simulink model "windEmulatorStep4_WECSim"  (R2025b)
settings: Solver=ode14x  StartTime=0  StopTime=400  FixedStep=Ts  MaxStep=0.01  RelTol=1e-3
values from neighbouring files (symbols this model uses):
  A = 1.0    (= 1)    [initStep4.m]
  absEncoderCountsToRad = 1/2^20*2*pi    (= 5.99211245268e-06)    [initStep4.m]
  acs800CtrlStruct =     [windEmulatorBusDefs.mat]
  acs800DcBusVoltsScaling = 1    [initStep4.m]
  acs800FreqScaling = 1/100    (= 0.01)    [initStep4.m]
  acs800PowerScaling = Gen_PowerScaling    (= 14.9109)    [initStep4.m]
  acs800SignalStruct =     [windEmulatorBusDefs.mat]
  acs800SpeedNomEng = 1500    [initStep4.m]
  acs800SpeedNomFb = 20000    [initStep4.m]
  acs800SpeedScaling = 1500/20000    (= 0.075)    [initStep4.m]
  acs800TempScaling = 1/10    (= 0.1)    [initStep4.m]
  acs800TorqueNomEng = 100    [initStep4.m]
  acs800TorqueNomFb = 10000    [initStep4.m]
  acs800TorqueScaling = acs800TorqueRating/10000    (= 0.008035933)    [initStep4.m]
  acs880CtrlStruct =     [windEmulatorBusDefs.mat]
  acs880FreqScaling = 60/20000    (= 0.003)    [initStep4.m]
  acs880MotorCurrentScaling = 100/10000    (= 0.01)    [initStep4.m]
  acs880MotorVoltsScaling = 1    [initStep4.m]
  acs880PowerScaling = 100*hp2W/10000    (= 7.457)    [initStep4.m]
  acs880RatedTorque = 80.494    [initStep4.m]
  acs880RateLimFalling = -10000    [initStep4.m]
  acs880RateLimRising = 10000    [initStep4.m]
  acs880SetpointLimLower = -0.975*acs880RatedTorque    (= -78.48165)    [initStep4.m]
  acs880SetpointLimUpper = 0.975*acs880RatedTorque    (= 78.48165)    [initStep4.m]
  acs880SignalStruct =     [windEmulatorBusDefs.mat]
  acs880SpeedPILimLo = -0.975*acs880RatedTorque    (= -78.48165)    [initStep4.m]
  acs880SpeedPILimUp = 0.975*acs880RatedTorque    (= 78.48165)    [initStep4.m]
  acs880SpeedScaling = 2000/20000    (= 0.1)    [initStep4.m]
  acs880TorqueFieldbusScale = 10000    [initStep4.m]
  acs880TorqueScaling = acs880RatedTorque/acs880TorqueFieldbusScale    (= 0.0080494)    [initStep4.m]
  acs880TorqueSetpointScaling = 100    [initStep4.m]
  bar2pa = 1e5    (= 100000)    [initStep4.m]
  belowMinPGain = 1/200    (= 0.005)    [initStep4.m]
  ctrlModeTorque = logical(true)    [init.m]    (also in initStep1.m; initStep2.m; initStep3.m; initStep4.m)
  ctrlSignal1 = squeeze(hptoSignalsData.Values.ctrlSignal1.Data)    [postProcessingStep2.m]
  ctrlSignal2 = squeeze(hptoSignalsData.Values.ctrlSignal2.Data)    [postProcessingStep2.m]
  deadBandController = boolean(false)    [initStep4.m]
  deadbandTorqueSlewRate = 300    [initStep4.m]
  Dm_max = 40    [initStep4.m]
  EffMechMax = 0.93    [initStep4.m]
  EffMechMin = 0.79    [initStep4.m]
  excForce_N = squeeze(hptoCtrlData.Values.excForce_N.Data)    [postProcessingStep2.m]
  expCtrlStruct =     [windEmulatorBusDefs.mat]
  FactorEff = psi2pa*cc2m3*(1/rev2rad)    (= 0.00109733470463)    [initStep4.m]
  fromFileSpeedSlewRate = 250    [initStep4.m]
  fromFileTorqueSlewRate = 25    [initStep4.m]
  futekTorqueScale = -1/(2^31)*10/5*100    (= -9.31322574615e-08)    [initStep4.m]
  genMaxTorque = 0.8*ratedTorque    (= 64.3952)    [initStep3.m]    (also in initStep4.m = 78.48165)
  genTorqueCmd_Nm = squeeze(hptoSignalsData.Values.genTorqueCmd_Nm.Data)    [postProcessingStep2.m]
  hbmCtScale = 1/1.5    (= 0.666666666667)    [initStep4.m]
  hbmPowerStruct =     [windEmulatorBusDefs.mat]
  hptoCtrlStruct =     [windEmulatorBusDefs.mat]
  hptoSignalStruct =     [windEmulatorBusDefs.mat]
  invPowerStruct =     [windEmulatorBusDefs.mat]
  lpm2m3ps = 1/m3ps2lpm    (= 1.66666666667e-05)    [initStep4.m]
  minPressureRef_psi = 1000    [initStep4.m]
  minTorqueRef_Nm = (minPressureRef_psi*psi2pa)*(Dm_max*cc2m3*(1/rev2rad))    (= 43.8933881851)    [initStep4.m]
  motorSpeed_rpm = squeeze(acs880SignalsData.Values.motorSpeed_rpm.Data)    [postProcessingStep2.m]
  nPreDrop = 2900    [initStep4.m]
  nPreDropMin = 725    [initStep4.m]
  psi2bar = 1/bar2psi    (= 0.0689475729318)    [initStep4.m]
  radps2rpm = 60/(2*pi)    (= 9.54929658551)    [initStep2.m]    (also in initStep4.m)
  rpm2radps = 2*pi/60    (= 0.10471975512)    [initStep4.m]
  runCounter = squeeze(hptoCtrlData.Values.runCounter.Data)    [postProcessingStep2.m]
  shaftSignalStruct =     [windEmulatorBusDefs.mat]
  sidCtrlStruct =     [windEmulatorBusDefs.mat]
  sidDataCaseCounter = sidData.experimentData.count    [initStep4.m]
  sidDataSpeed_rpm = sidData.experimentData.wShaft_rpm    [initStep4.m]
  sidDataTorque_Nm = sidData.experimentData.torqueShaft_Nm    [initStep4.m]
  sidInfoStruct =     [windEmulatorBusDefs.mat]
  T = 4    [initStep4.m]
  targetOmega = 2000/60*2*pi    (= 209.439510239)    [initStep2.m]    (also in initStep3.m; initStep4.m)
  time = hptoCtrlData.Values.runCounter.Time    [postProcessingStep2.m]
  TorqueLoadMax = 75    [initStep4.m]
  Ts = 1/250    (= 0.004)    [initStep4.m]
undefined symbols (not defined in the file or in its folder): absEncoderCounts, absEncoderPosition_rad, absEncoderSpeed_rpm, absEncoderStatus1, absEncoderStatus2, absEncoderTurns, accVolHP, acs800Torque_Nm, acs800TorqueSetpoint_Nm, acs880SpeedSetpoint_rpm, acs880Torque_Nm, body, constraint, crankLength, ctrlWord, dcBusVoltage_V, DiscIntNeverNeededParam, Dmax, excShaftSpeed_rpm, excShaftTorque_Nm, expType, expTypeEnum, frequency_Hz, fromFileCaseCounter, genPumpFlow_lpm, genShaftSpeed_rpm, genShaftSpeedRef, genSpeedActual, hmOutputShafTorque_Nm, iGainGen, m3persecond2lpm, motorCurrent_A, motorTorque_Nm, motorVoltage_V, offsetLength, pa2psi, pGainGen, pressure_bar, PressureControl, pto, radsec2rpm, ramp, resetHilIntegrator, resetSidIntegrator, rodLength, runHil, runSid, shaftPower_W, sidType, sidTypeEnum, SpeedControl, speedCtrlReset, speedRef_rpm, state, statusWord, stepCounter, temperature, torqueActual_Nm, TorqueInputControl, torqueSetpoint_Nm ... (+1)
libraries: slrealtimeethercatlib x118, fl_lib x81, nesl_utility x45, sh_lib x18, slrealtimeloglib x13, dspstat3 x5, slpidlib x4, simulink_extras x4, cstblocks x3, dspindex x3, WECSim_Lib_Body_Elements x2, simulink x2
(part 5 of 6)

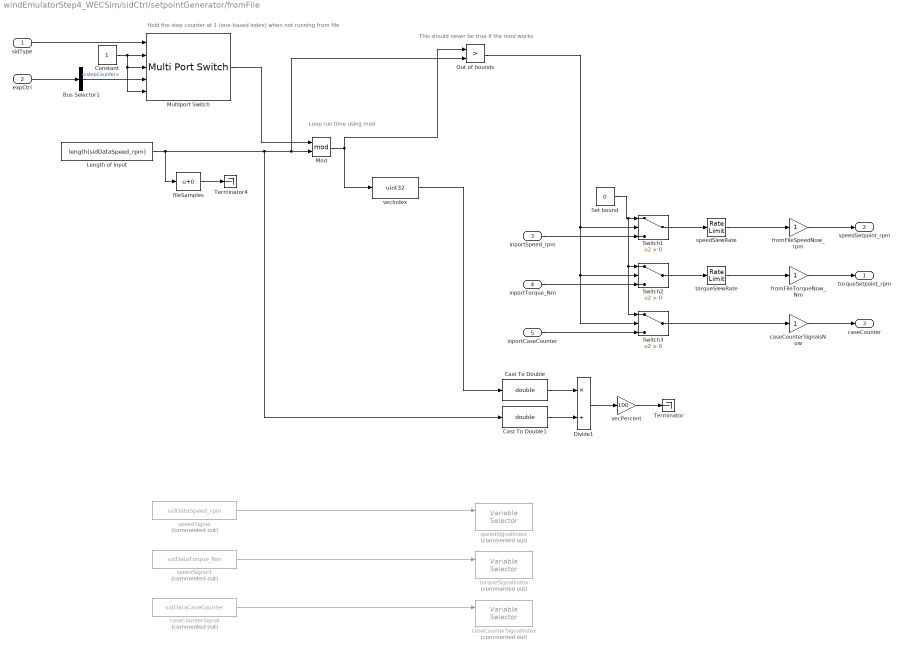
== system windEmulatorStep4_WECSim/sidCtrl/setpointGenerator/fromFile ==
  note: Hold the step counter at 1 (one-based index) when not running from file
  note: This should never be true if the mod works
  note: Loop run time using mod
  sidType : Inport  OutDataTypeStr=Enum: sidTypeEnum
  expCtrl : Inport  Port=2  OutDataTypeStr=Bus: expCtrlBus
  inportSpeed_rpm : Inport  Port=3
  inportTorque_Nm : Inport  Port=4
  inportCaseCounter : Inport  Port=5
  Bus Selector1 : BusSelector  OutputSignals=stepCounter
  Cast To Double : DataTypeConversion  OutDataTypeStr=double  SaturateOnIntegerOverflow=off  RndMeth=Floor
  Cast To Double1 : DataTypeConversion  OutDataTypeStr=double  SaturateOnIntegerOverflow=off  RndMeth=Floor
  Constant : Constant  OutDataTypeStr=uint32
  Divide1 : Product  Inputs=*/
  Length of input : Constant  Value=length(sidDataSpeed_rpm)  OutDataTypeStr=uint32
  Mod : Math  Operator=mod
  Multiport Switch : MultiPortSwitch  DataPortOrder=Specify indices  DataPortIndices={sidTypeEnum.off,sidTypeEnum.manual,sidTypeEnum.fromFile}  DataPortForDefault=Additional data port  SaturateOnIntegerOverflow=off  InputSameDT=off
  Out of bounds : RelationalOperator  Operator=>  OutDataTypeStr=boolean  RndMeth=Simplest  InputSameDT=off
  Set bound : Constant  Value=0
  Switch1 : Switch  Criteria=u2 > Threshold  SaturateOnIntegerOverflow=off  InputSameDT=off
  Switch2 : Switch  Criteria=u2 > Threshold  SaturateOnIntegerOverflow=off  InputSameDT=off
  Switch3 : Switch  Criteria=u2 > Threshold  SaturateOnIntegerOverflow=off  InputSameDT=off
  Terminator : Terminator
  Terminator4 : Terminator
  caseCounterSignal : Constant  Commented=on  Value=sidDataCaseCounter
  caseCounterSignalIndex : dspindex/Variable Selector  Commented=on  NumInputs=1  rowsOrCols=Columns  IdxMode=Variable  Elements=[1 3]  ZerOneIdxMode=One-based  errmode=Clip and Warn  FillMode=on  FillValues=0
  caseCounterSignalsNow : Gain
  fileSamples : Bias  SaturateOnIntegerOverflow=off
  fromFileSpeedNow_rpm : Gain
  fromFileTorqueNow_Nm : Gain
  speedSignal : Constant  Commented=on  Value=sidDataSpeed_rpm
  speedSignal1 : Constant  Commented=on  Value=sidDataTorque_Nm
  speedSignalIndex : dspindex/Variable Selector  Commented=on  NumInputs=1  rowsOrCols=Columns  IdxMode=Variable  Elements=[1 3]  ZerOneIdxMode=One-based  errmode=Clip and Warn  FillMode=on  FillValues=0
  speedSlewRate : RateLimiter  RisingSlewLimit=fromFileSpeedSlewRate  FallingSlewLimit=-fromFileSpeedSlewRate  SampleTimeMode=inherited
  torqueSignalIndex : dspindex/Variable Selector  Commented=on  NumInputs=1  rowsOrCols=Columns  IdxMode=Variable  Elements=[1 3]  ZerOneIdxMode=One-based  errmode=Clip and Warn  FillMode=on  FillValues=0
  torqueSlewRate : RateLimiter  RisingSlewLimit=fromFileTorqueSlewRate  FallingSlewLimit=-fromFileTorqueSlewRate  SampleTimeMode=inherited
  vecIndex : DataTypeConversion  OutDataTypeStr=uint32  SaturateOnIntegerOverflow=off  RndMeth=Floor
  vecPercent : Gain  Gain=100
  torqueSetpoint_rpm : Outport
  speedSetpoint_rpm : Outport  Port=2
  caseCounter : Outport  Port=3
  wires:
  vecPercent/1 -> Terminator/1
  Cast To Double/1 -> Divide1/1
  Length of input/1 -> Cast To Double1/1, Out of bounds/2, Mod/2, fileSamples/1
  fromFileTorqueNow_Nm/1 -> torqueSetpoint_rpm/1
  speedSignal/1 -> speedSignalIndex/1
  Out of bounds/1 -> Switch3/2, Switch2/2, Switch1/2
  torqueSlewRate/1 -> fromFileTorqueNow_Nm/1
  caseCounterSignal/1 -> caseCounterSignalIndex/1
  Switch2/1 -> torqueSlewRate/1
  speedSlewRate/1 -> fromFileSpeedNow_rpm/1
  vecIndex/1 -> Cast To Double/1
  Set bound/1 -> Switch2/1, Switch3/1, Switch1/1
  Switch1/1 -> speedSlewRate/1
  Mod/1 -> vecIndex/1, Out of bounds/1
  fileSamples/1 -> Terminator4/1
  Divide1/1 -> vecPercent/1
  caseCounterSignalsNow/1 -> caseCounter/1
  Switch3/1 -> caseCounterSignalsNow/1
  fromFileSpeedNow_rpm/1 -> speedSetpoint_rpm/1
  Cast To Double1/1 -> Divide1/2
  expCtrl/1 -> Bus Selector1/1
  speedSignal1/1 -> torqueSignalIndex/1
  sidType/1 -> Multiport Switch/1
  Bus Selector1/1 -> Multiport Switch/4  "<stepCounter>"
  Multiport Switch/1 -> Mod/1
  Constant/1 -> Multiport Switch/5, Multiport Switch/3, Multiport Switch/2
  inportSpeed_rpm/1 -> Switch1/3
  inportTorque_Nm/1 -> Switch2/3
  inportCaseCounter/1 -> Switch3/3

== system windEmulatorStep4_WECSim/hptoSim/WECSimModel/Subsystem/Angular to Linear Velocity ==
  angPos : Inport
  angVel : Inport  Port=2
  Add1 : Sum  Inputs=+-
  Add2 : Sum  Inputs=+-
  Add5 : Sum  Inputs=+-
  Add7 : Sum
  Constant1 : Constant  Value=rodLength
  Constant{2,5,8..9} (4 alike) : Constant  Value=crankLength
  Constant3 : Constant  Value=offsetLength
  Constant6 : Constant  Value=offsetLength
  Divide1 : Product  Inputs=*/
  Math Function1 : Math  Operator=square  SignedPower=on
  Math Function2 : Math  Operator=square  SignedPower=on
  Product1 : Product  Inputs=**
  Product5 : Product  Inputs=**
  Product6 : Product  Inputs=***
  Product8 : Product  Inputs=***
  Product9 : Product  Inputs=**
  Sqrt2 : Sqrt
  Trigonometric Function1 : Trigonometry  Operator=cos
  Trigonometric Function3 : Trigonometry  Operator=cos
  Trigonometric Function4 : Trigonometry  Operator=cos
  Trigonometric Function6 : Trigonometry
  linearVel : Outport
  wires:
  Math Function2/1 -> Add1/1
  Divide1/1 -> Add7/2
  Product8/1 -> Divide1/1
  Sqrt2/1 -> Divide1/2
  Math Function1/1 -> Add1/2
  Constant1/1 -> Math Function2/1
  Constant3/1 -> Add2/2
  Product1/1 -> Add2/1
  Trigonometric Function1/1 -> Product1/2
  Constant2/1 -> Product1/1
  Add1/1 -> Sqrt2/1
  Add2/1 -> Math Function1/1
  angPos/1 -> Trigonometric Function4/1, Trigonometric Function3/1, Trigonometric Function6/1, Trigonometric Function1/1
  Product9/1 -> Product8/3
  Add5/1 -> Product8/2
  angVel/1 -> Product6/3, Product8/1
  Trigonometric Function6/1 -> Product9/2
  Constant9/1 -> Product9/1
  Constant6/1 -> Add5/2
  Product5/1 -> Add5/1
  Trigonometric Function3/1 -> Product5/2
  Constant5/1 -> Product5/1
  Product6/1 -> Add7/1
  Constant8/1 -> Product6/1
  Trigonometric Function4/1 -> Product6/2
  Add7/1 -> linearVel/1

== system windEmulatorStep4_WECSim/hptoSim/WECSimModel/Subsystem/FlowSensor1 ==
  Gain : Gain  Gain=m3persecond2lpm
  Hydraulic Flow Rate Sensor : fl_lib/Hydraulic/Hydraulic Sensors/Hydraulic Flow Rate Sensor
  PS Terminator : fl_lib/Physical Signals/Sinks/PS Terminator
  PS-Simulink Converter2 : nesl_utility/PS-Simulink Converter  PhysicalDomain=network_engine_domain  SubClassName=ps_output  LeftPortType=input  RightPortType=output  PseudoPeriodic=off  Frequencies=[]  VectorFormat=inherit  Unit=inherit  AffineConversion=off
  Terminator : Terminator
  B : PMIOPort  Side=Right
  A : PMIOPort  Port=2  Side=Left
  wires:
  PS-Simulink Converter2/1 -> Gain/1
  Gain/1 -> Terminator/1  "flowRateHCB"
  connections:
  Hydraulic Flow Rate Sensor/LConn1 -- A/RConn1
  PS Terminator/LConn1 -- Hydraulic Flow Rate Sensor/RConn3
  PS-Simulink Converter2/LConn1 -- Hydraulic Flow Rate Sensor/RConn1
  Hydraulic Flow Rate Sensor/RConn2 -- B/RConn1

== system windEmulatorStep4_WECSim/hptoSim/WECSimModel/Subsystem/FlowSensor10 ==
  Gain : Gain  Gain=m3persecond2lpm
  Hydraulic Flow Rate Sensor : fl_lib/Hydraulic/Hydraulic Sensors/Hydraulic Flow Rate Sensor
  PS Terminator : fl_lib/Physical Signals/Sinks/PS Terminator
  PS-Simulink Converter2 : nesl_utility/PS-Simulink Converter  PhysicalDomain=network_engine_domain  SubClassName=ps_output  LeftPortType=input  RightPortType=output  PseudoPeriodic=off  Frequencies=[]  VectorFormat=inherit  Unit=inherit  AffineConversion=off
  Terminator : Terminator
  B : PMIOPort  Side=Right
  A : PMIOPort  Port=2  Side=Left
  wires:
  PS-Simulink Converter2/1 -> Gain/1
  Gain/1 -> Terminator/1  "flowRateCV4"
  connections:
  Hydraulic Flow Rate Sensor/LConn1 -- A/RConn1
  PS Terminator/LConn1 -- Hydraulic Flow Rate Sensor/RConn3
  PS-Simulink Converter2/LConn1 -- Hydraulic Flow Rate Sensor/RConn1
  Hydraulic Flow Rate Sensor/RConn2 -- B/RConn1

== system windEmulatorStep4_WECSim/hptoSim/WECSimModel/Subsystem/FlowSensor13 ==
  Gain : Gain  Gain=m3persecond2lpm
  Hydraulic Flow Rate Sensor : fl_lib/Hydraulic/Hydraulic Sensors/Hydraulic Flow Rate Sensor
  PS Terminator : fl_lib/Physical Signals/Sinks/PS Terminator
  PS-Simulink Converter2 : nesl_utility/PS-Simulink Converter  PhysicalDomain=network_engine_domain  SubClassName=ps_output  LeftPortType=input  RightPortType=output  PseudoPeriodic=off  Frequencies=[]  VectorFormat=inherit  Unit=inherit  AffineConversion=off
  Terminator : Terminator
  B : PMIOPort  Side=Right
  A : PMIOPort  Port=2  Side=Left
  wires:
  PS-Simulink Converter2/1 -> Gain/1
  Gain/1 -> Terminator/1  "flowRateCV1"
  connections:
  Hydraulic Flow Rate Sensor/LConn1 -- A/RConn1
  PS Terminator/LConn1 -- Hydraulic Flow Rate Sensor/RConn3
  PS-Simulink Converter2/LConn1 -- Hydraulic Flow Rate Sensor/RConn1
  Hydraulic Flow Rate Sensor/RConn2 -- B/RConn1

== system windEmulatorStep4_WECSim/hptoSim/WECSimModel/Subsystem/FlowSensor16 ==
  Gain : Gain  Gain=m3persecond2lpm
  Hydraulic Flow Rate Sensor : fl_lib/Hydraulic/Hydraulic Sensors/Hydraulic Flow Rate Sensor
  PS Terminator : fl_lib/Physical Signals/Sinks/PS Terminator
  PS-Simulink Converter2 : nesl_utility/PS-Simulink Converter  PhysicalDomain=network_engine_domain  SubClassName=ps_output  LeftPortType=input  RightPortType=output  PseudoPeriodic=off  Frequencies=[]  VectorFormat=inherit  Unit=inherit  AffineConversion=off
  Terminator : Terminator
  B : PMIOPort  Side=Right
  A : PMIOPort  Port=2  Side=Left
  wires:
  PS-Simulink Converter2/1 -> Gain/1
  Gain/1 -> Terminator/1  "flowRateCV3"
  connections:
  Hydraulic Flow Rate Sensor/LConn1 -- A/RConn1
  PS Terminator/LConn1 -- Hydraulic Flow Rate Sensor/RConn3
  PS-Simulink Converter2/LConn1 -- Hydraulic Flow Rate Sensor/RConn1
  Hydraulic Flow Rate Sensor/RConn2 -- B/RConn1

== system windEmulatorStep4_WECSim/hptoSim/WECSimModel/Subsystem/FlowSensor2 ==
  Gain : Gain  Gain=m3persecond2lpm
  Hydraulic Flow Rate Sensor : fl_lib/Hydraulic/Hydraulic Sensors/Hydraulic Flow Rate Sensor
  PS Terminator : fl_lib/Physical Signals/Sinks/PS Terminator
  PS-Simulink Converter2 : nesl_utility/PS-Simulink Converter  PhysicalDomain=network_engine_domain  SubClassName=ps_output  LeftPortType=input  RightPortType=output  PseudoPeriodic=off  Frequencies=[]  VectorFormat=inherit  Unit=inherit  AffineConversion=off
  Terminator : Terminator
  B : PMIOPort  Side=Right
  A : PMIOPort  Port=2  Side=Left
  wires:
  PS-Simulink Converter2/1 -> Gain/1
  Gain/1 -> Terminator/1  "flowRateHCA"
  connections:
  Hydraulic Flow Rate Sensor/LConn1 -- A/RConn1
  PS Terminator/LConn1 -- Hydraulic Flow Rate Sensor/RConn3
  PS-Simulink Converter2/LConn1 -- Hydraulic Flow Rate Sensor/RConn1
  Hydraulic Flow Rate Sensor/RConn2 -- B/RConn1

== system windEmulatorStep4_WECSim/hptoSim/WECSimModel/Subsystem/FlowSensor3 ==
  Gain : Gain  Gain=m3persecond2lpm
  Hydraulic Flow Rate Sensor : fl_lib/Hydraulic/Hydraulic Sensors/Hydraulic Flow Rate Sensor
  PS Terminator : fl_lib/Physical Signals/Sinks/PS Terminator
  PS-Simulink Converter2 : nesl_utility/PS-Simulink Converter  PhysicalDomain=network_engine_domain  SubClassName=ps_output  LeftPortType=input  RightPortType=output  PseudoPeriodic=off  Frequencies=[]  VectorFormat=inherit  Unit=inherit  AffineConversion=off
  Terminator : Terminator
  B : PMIOPort  Side=Right
  A : PMIOPort  Port=2  Side=Left
  wires:
  PS-Simulink Converter2/1 -> Gain/1
  Gain/1 -> Terminator/1  "flowRateC"
  connections:
  Hydraulic Flow Rate Sensor/LConn1 -- A/RConn1
  PS Terminator/LConn1 -- Hydraulic Flow Rate Sensor/RConn3
  PS-Simulink Converter2/LConn1 -- Hydraulic Flow Rate Sensor/RConn1
  Hydraulic Flow Rate Sensor/RConn2 -- B/RConn1

== system windEmulatorStep4_WECSim/hptoSim/WECSimModel/Subsystem/FlowSensor4 ==
  Gain : Gain  Gain=m3persecond2lpm
  Hydraulic Flow Rate Sensor : fl_lib/Hydraulic/Hydraulic Sensors/Hydraulic Flow Rate Sensor
  PS Terminator : fl_lib/Physical Signals/Sinks/PS Terminator
  PS-Simulink Converter2 : nesl_utility/PS-Simulink Converter  PhysicalDomain=network_engine_domain  SubClassName=ps_output  LeftPortType=input  RightPortType=output  PseudoPeriodic=off  Frequencies=[]  VectorFormat=inherit  Unit=inherit  AffineConversion=off
  Terminator : Terminator
  B : PMIOPort  Side=Right
  A : PMIOPort  Port=2  Side=Left
  wires:
  PS-Simulink Converter2/1 -> Gain/1
  Gain/1 -> Terminator/1  "flowRateAccHP"
  connections:
  Hydraulic Flow Rate Sensor/LConn1 -- A/RConn1
  PS Terminator/LConn1 -- Hydraulic Flow Rate Sensor/RConn3
  PS-Simulink Converter2/LConn1 -- Hydraulic Flow Rate Sensor/RConn1
  Hydraulic Flow Rate Sensor/RConn2 -- B/RConn1

== system windEmulatorStep4_WECSim/hptoSim/WECSimModel/Subsystem/FlowSensor5 ==
  Gain : Gain  Gain=m3persecond2lpm
  Hydraulic Flow Rate Sensor : fl_lib/Hydraulic/Hydraulic Sensors/Hydraulic Flow Rate Sensor
  PS Terminator : fl_lib/Physical Signals/Sinks/PS Terminator
  PS-Simulink Converter2 : nesl_utility/PS-Simulink Converter  PhysicalDomain=network_engine_domain  SubClassName=ps_output  LeftPortType=input  RightPortType=output  PseudoPeriodic=off  Frequencies=[]  VectorFormat=inherit  Unit=inherit  AffineConversion=off
  Terminator : Terminator
  B : PMIOPort  Side=Right
  A : PMIOPort  Port=2  Side=Left
  wires:
  PS-Simulink Converter2/1 -> Gain/1
  Gain/1 -> Terminator/1  "flowRateHMin"
  connections:
  Hydraulic Flow Rate Sensor/LConn1 -- A/RConn1
  PS Terminator/LConn1 -- Hydraulic Flow Rate Sensor/RConn3
  PS-Simulink Converter2/LConn1 -- Hydraulic Flow Rate Sensor/RConn1
  Hydraulic Flow Rate Sensor/RConn2 -- B/RConn1

== system windEmulatorStep4_WECSim/hptoSim/WECSimModel/Subsystem/FlowSensor6 ==
  Gain : Gain  Gain=m3persecond2lpm
  Hydraulic Flow Rate Sensor : fl_lib/Hydraulic/Hydraulic Sensors/Hydraulic Flow Rate Sensor
  PS Terminator : fl_lib/Physical Signals/Sinks/PS Terminator
  PS-Simulink Converter2 : nesl_utility/PS-Simulink Converter  PhysicalDomain=network_engine_domain  SubClassName=ps_output  LeftPortType=input  RightPortType=output  PseudoPeriodic=off  Frequencies=[]  VectorFormat=inherit  Unit=inherit  AffineConversion=off
  Terminator : Terminator
  B : PMIOPort  Side=Right
  A : PMIOPort  Port=2  Side=Left
  wires:
  PS-Simulink Converter2/1 -> Gain/1
  Gain/1 -> Terminator/1  "flowRateHMout"
  connections:
  Hydraulic Flow Rate Sensor/LConn1 -- A/RConn1
  PS Terminator/LConn1 -- Hydraulic Flow Rate Sensor/RConn3
  PS-Simulink Converter2/LConn1 -- Hydraulic Flow Rate Sensor/RConn1
  Hydraulic Flow Rate Sensor/RConn2 -- B/RConn1

== system windEmulatorStep4_WECSim/hptoSim/WECSimModel/Subsystem/FlowSensor7 ==
  Gain : Gain  Gain=m3persecond2lpm
  Hydraulic Flow Rate Sensor : fl_lib/Hydraulic/Hydraulic Sensors/Hydraulic Flow Rate Sensor
  PS Terminator : fl_lib/Physical Signals/Sinks/PS Terminator
  PS-Simulink Converter2 : nesl_utility/PS-Simulink Converter  PhysicalDomain=network_engine_domain  SubClassName=ps_output  LeftPortType=input  RightPortType=output  PseudoPeriodic=off  Frequencies=[]  VectorFormat=inherit  Unit=inherit  AffineConversion=off
  Terminator : Terminator
  B : PMIOPort  Side=Right
  A : PMIOPort  Port=2  Side=Left
  wires:
  PS-Simulink Converter2/1 -> Gain/1
  Gain/1 -> Terminator/1  "flowRateAccLP"
  connections:
  Hydraulic Flow Rate Sensor/LConn1 -- A/RConn1
  PS Terminator/LConn1 -- Hydraulic Flow Rate Sensor/RConn3
  PS-Simulink Converter2/LConn1 -- Hydraulic Flow Rate Sensor/RConn1
  Hydraulic Flow Rate Sensor/RConn2 -- B/RConn1

== system windEmulatorStep4_WECSim/hptoSim/WECSimModel/Subsystem/FlowSensor8 ==
  Gain : Gain  Gain=m3persecond2lpm
  Hydraulic Flow Rate Sensor : fl_lib/Hydraulic/Hydraulic Sensors/Hydraulic Flow Rate Sensor
  PS Terminator : fl_lib/Physical Signals/Sinks/PS Terminator
  PS-Simulink Converter2 : nesl_utility/PS-Simulink Converter  PhysicalDomain=network_engine_domain  SubClassName=ps_output  LeftPortType=input  RightPortType=output  PseudoPeriodic=off  Frequencies=[]  VectorFormat=inherit  Unit=inherit  AffineConversion=off
  Terminator : Terminator
  B : PMIOPort  Side=Right
  A : PMIOPort  Port=2  Side=Left
  wires:
  PS-Simulink Converter2/1 -> Gain/1
  Gain/1 -> Terminator/1  "flowRateD"
  connections:
  Hydraulic Flow Rate Sensor/LConn1 -- A/RConn1
  PS Terminator/LConn1 -- Hydraulic Flow Rate Sensor/RConn3
  PS-Simulink Converter2/LConn1 -- Hydraulic Flow Rate Sensor/RConn1
  Hydraulic Flow Rate Sensor/RConn2 -- B/RConn1

== system windEmulatorStep4_WECSim/hptoSim/WECSimModel/Subsystem/FlowSensor9 ==
  Gain : Gain  Gain=m3persecond2lpm
  Hydraulic Flow Rate Sensor : fl_lib/Hydraulic/Hydraulic Sensors/Hydraulic Flow Rate Sensor
  PS Terminator : fl_lib/Physical Signals/Sinks/PS Terminator
  PS-Simulink Converter2 : nesl_utility/PS-Simulink Converter  PhysicalDomain=network_engine_domain  SubClassName=ps_output  LeftPortType=input  RightPortType=output  PseudoPeriodic=off  Frequencies=[]  VectorFormat=inherit  Unit=inherit  AffineConversion=off
  Terminator : Terminator
  B : PMIOPort  Side=Right
  A : PMIOPort  Port=2  Side=Left
  wires:
  PS-Simulink Converter2/1 -> Gain/1
  Gain/1 -> Terminator/1  "flowRateCV2"
  connections:
  Hydraulic Flow Rate Sensor/LConn1 -- A/RConn1
  PS Terminator/LConn1 -- Hydraulic Flow Rate Sensor/RConn3
  PS-Simulink Converter2/LConn1 -- Hydraulic Flow Rate Sensor/RConn1
  Hydraulic Flow Rate Sensor/RConn2 -- B/RConn1

== system windEmulatorStep4_WECSim/hptoSim/WECSimModel/Subsystem/pistonPosition ==
  Ideal Translational Motion Sensor : fl_lib/Mechanical/Mechanical Sensors/Ideal Translational Motion Sensor  reference=foundation.enum.MeasurementReference.difference  acceleration_port=false  velocity_port=true  position_port=true  offset=0 m
  Mechanical Translational Reference1 : fl_lib/Mechanical/Translational Elements/Mechanical Translational Reference
  PS Terminator : fl_lib/Physical Signals/Sinks/PS Terminator
  PS-Simulink Converter : nesl_utility/PS-Simulink Converter  PhysicalDomain=network_engine_domain  SubClassName=ps_output  LeftPortType=input  RightPortType=output  PseudoPeriodic=off  Frequencies=[]  VectorFormat=inherit  Unit=inherit  AffineConversion=off
  PS-Simulink Converter2 : nesl_utility/PS-Simulink Converter  PhysicalDomain=network_engine_domain  SubClassName=ps_output  LeftPortType=input  RightPortType=output  PseudoPeriodic=off  Frequencies=[]  VectorFormat=inherit  Unit=inherit  AffineConversion=off
  Scope : Scope
      settings: ActiveDisplayYMinimum=-0.080911717849368445  ActiveDisplayYMaximum=0.6625292550148727  DataLoggingVariableName=ScopeData5
  Terminator : Terminator
  Conn1 : PMIOPort  Side=Left
  Out1 : Outport
  wires:
  PS-Simulink Converter2/1 -> Scope/1, Terminator/1  "pistonPosition"
  PS-Simulink Converter/1 -> Out1/1
  connections:
  Ideal Translational Motion Sensor/LConn1 -- Conn1/RConn1
  PS Terminator/LConn1 -- PS-Simulink Converter/LConn1 -- Ideal Translational Motion Sensor/RConn2
  PS-Simulink Converter2/LConn1 -- Ideal Translational Motion Sensor/RConn3
  Mechanical Translational Reference1/LConn1 -- Ideal Translational Motion Sensor/RConn1

== system windEmulatorStep4_WECSim/hptoSim/WECSimModel/Subsystem/pressureSensorA ==
  Gain : Gain  Gain=pa2psi
  Hydraulic Pressure Sensor : fl_lib/Hydraulic/Hydraulic Sensors/Hydraulic Pressure Sensor
  Hydraulic Reference : fl_lib/Hydraulic/Hydraulic Elements/Hydraulic Reference
  PS-Simulink Converter2 : nesl_utility/PS-Simulink Converter  PhysicalDomain=network_engine_domain  SubClassName=ps_output  LeftPortType=input  RightPortType=output  PseudoPeriodic=off  Frequencies=[]  VectorFormat=inherit  Unit=inherit  AffineConversion=off
  Scope : Scope
      settings: ActiveDisplayYMinimum=-108.18611715828341  ActiveDisplayYMaximum=973.67505442455092  DataLoggingVariableName=ScopeData4
  Terminator : Terminator
  Conn1 : PMIOPort  Side=Left
  wires:
  Gain/1 -> Scope/1, Terminator/1  "pressureA"
  PS-Simulink Converter2/1 -> Gain/1
  connections:
  PS-Simulink Converter2/LConn1 -- Hydraulic Pressure Sensor/RConn2
  Hydraulic Reference/LConn1 -- Hydraulic Pressure Sensor/RConn1
  Hydraulic Pressure Sensor/LConn1 -- Conn1/RConn1

== system windEmulatorStep4_WECSim/hptoSim/WECSimModel/Subsystem/pressureSensorB ==
  Gain : Gain  Gain=pa2psi
  Hydraulic Pressure Sensor : fl_lib/Hydraulic/Hydraulic Sensors/Hydraulic Pressure Sensor
  Hydraulic Reference : fl_lib/Hydraulic/Hydraulic Elements/Hydraulic Reference
  PS-Simulink Converter2 : nesl_utility/PS-Simulink Converter  PhysicalDomain=network_engine_domain  SubClassName=ps_output  LeftPortType=input  RightPortType=output  PseudoPeriodic=off  Frequencies=[]  VectorFormat=inherit  Unit=inherit  AffineConversion=off
  Scope : Scope
      settings: ActiveDisplayYMinimum=-22.167205478263213  ActiveDisplayYMaximum=1755.5061383660914  DataLoggingVariableName=ScopeData3
  Terminator : Terminator
  Conn1 : PMIOPort  Side=Left
  wires:
  Gain/1 -> Scope/1, Terminator/1  "pressureB"
  PS-Simulink Converter2/1 -> Gain/1
  connections:
  PS-Simulink Converter2/LConn1 -- Hydraulic Pressure Sensor/RConn2
  Hydraulic Reference/LConn1 -- Hydraulic Pressure Sensor/RConn1
  Hydraulic Pressure Sensor/LConn1 -- Conn1/RConn1

== system windEmulatorStep4_WECSim/hptoSim/WECSimModel/Subsystem/pressureSensorC ==
  Gain : Gain  Gain=pa2psi
  Hydraulic Pressure Sensor : fl_lib/Hydraulic/Hydraulic Sensors/Hydraulic Pressure Sensor
  Hydraulic Reference : fl_lib/Hydraulic/Hydraulic Elements/Hydraulic Reference
  PS-Simulink Converter2 : nesl_utility/PS-Simulink Converter  PhysicalDomain=network_engine_domain  SubClassName=ps_output  LeftPortType=input  RightPortType=output  PseudoPeriodic=off  Frequencies=[]  VectorFormat=inherit  Unit=inherit  AffineConversion=off
  Terminator : Terminator
  Conn1 : PMIOPort  Side=Left
  wires:
  Gain/1 -> Terminator/1  "pressureC"
  PS-Simulink Converter2/1 -> Gain/1
  connections:
  PS-Simulink Converter2/LConn1 -- Hydraulic Pressure Sensor/RConn2
  Hydraulic Reference/LConn1 -- Hydraulic Pressure Sensor/RConn1
  Hydraulic Pressure Sensor/LConn1 -- Conn1/RConn1

== system windEmulatorStep4_WECSim/hptoSim/WECSimModel/Subsystem/pressureSensorC1 ==
  Gain : Gain  Gain=pa2psi
  Hydraulic Pressure Sensor : fl_lib/Hydraulic/Hydraulic Sensors/Hydraulic Pressure Sensor
  Hydraulic Reference : fl_lib/Hydraulic/Hydraulic Elements/Hydraulic Reference
  PS-Simulink Converter2 : nesl_utility/PS-Simulink Converter  PhysicalDomain=network_engine_domain  SubClassName=ps_output  LeftPortType=input  RightPortType=output  PseudoPeriodic=off  Frequencies=[]  VectorFormat=inherit  Unit=inherit  AffineConversion=off
  Scope : Scope
      settings: ActiveDisplayYMinimum=129.86941769572641  ActiveDisplayYMaximum=1541.1272657005441  DataLoggingVariableName=ScopeData6
  Terminator : Terminator
  Conn1 : PMIOPort  Side=Left
  wires:
  Gain/1 -> Scope/1, Terminator/1  "pressureHM"
  PS-Simulink Converter2/1 -> Gain/1
  connections:
  PS-Simulink Converter2/LConn1 -- Hydraulic Pressure Sensor/RConn2
  Hydraulic Reference/LConn1 -- Hydraulic Pressure Sensor/RConn1
  Hydraulic Pressure Sensor/LConn1 -- Conn1/RConn1

== system windEmulatorStep4_WECSim/hptoSim/WECSimModel/Subsystem/pressureSensorD ==
  Gain : Gain  Gain=pa2psi
  Hydraulic Pressure Sensor : fl_lib/Hydraulic/Hydraulic Sensors/Hydraulic Pressure Sensor
  Hydraulic Reference : fl_lib/Hydraulic/Hydraulic Elements/Hydraulic Reference
  PS-Simulink Converter2 : nesl_utility/PS-Simulink Converter  PhysicalDomain=network_engine_domain  SubClassName=ps_output  LeftPortType=input  RightPortType=output  PseudoPeriodic=off  Frequencies=[]  VectorFormat=inherit  Unit=inherit  AffineConversion=off
  Scope : Scope
      settings: ActiveDisplayYMinimum=-6.2082719103911472  ActiveDisplayYMaximum=137.72426049135703  DataLoggingVariableName=ScopeData7
  Terminator : Terminator
  Conn1 : PMIOPort  Side=Left
  wires:
  Gain/1 -> Scope/1, Terminator/1  "pressureD"
  PS-Simulink Converter2/1 -> Gain/1
  connections:
  PS-Simulink Converter2/LConn1 -- Hydraulic Pressure Sensor/RConn2
  Hydraulic Reference/LConn1 -- Hydraulic Pressure Sensor/RConn1
  Hydraulic Pressure Sensor/LConn1 -- Conn1/RConn1

== system windEmulatorStep4_WECSim/hptoSim/hptoModel/ControlAlgorithm/ForceToTorque ==
  ActualSignals : Inport
  Bus Selector : BusSelector  OutputSignals=LinearSpeedInput,LinearPositionInput
  Constant2 : Constant  Value=(A*2*pi/T)/targetOmega
  DesiredForce : Subsystem
  Gain : Gain  Gain=-1
  Product2 : Product
  TorqueD : Outport
  wires:
  ActualSignals/1 -> Bus Selector/1
  Product2/1 -> Gain/1
  Constant2/1 -> Product2/2
  Bus Selector/1 -> DesiredForce/1(<LinearSpeedInput>)  "<LinearSpeedInput>"
  Bus Selector/2 -> DesiredForce/2(<LinearPositionInput>)  "<LinearPositionInput>"
  DesiredForce/1(ForceD) -> Product2/1
  Gain/1 -> TorqueD/1

== system windEmulatorStep4_WECSim/hptoSim/hptoModel/ControlAlgorithm/PressureAbovePmin ==
  ActualSignals : Inport
  RefValues : Inport  Port=2
  SpeedControllerReset : Inport  Port=3
  Bus Selector : BusSelector  OutputSignals=TorqueShaftInput,Pressure,wShaft
  Bus Selector1 : BusSelector  OutputSignals=TorqueInputRef,PressureRef,SheftSpeedRef
  PressureControl1 : Subsystem
  SpeedControl1 : Subsystem
  Terminator1 : Terminator
  TorqueControl1 : Subsystem
  ControlSignal1 : Outport
  ControlSignal2 : Outport  Port=2
  ControlTorqueLoad : Outport  Port=3
  wires:
  ActualSignals/1 -> Bus Selector/1
  TorqueControl1/1(ControlSignal1) -> ControlSignal1/1
  Bus Selector/3 -> SpeedControl1/1(ShaftSpeedMotor)  "<wShaft>"
  RefValues/1 -> Bus Selector1/1
  Bus Selector1/1 -> TorqueControl1/1(TorqueRef)  "<TorqueInputRef>"
  Bus Selector1/3 -> SpeedControl1/2(ShaftSpeedRef)  "<SheftSpeedRef>"
  PressureControl1/1(ControlSignal2) -> ControlSignal2/1
  Bus Selector/2 -> PressureControl1/1(ActualPressure)  "<Pressure>"
  Bus Selector/1 -> Terminator1/1  "<TorqueShaftInput>"
  Bus Selector1/2 -> PressureControl1/2(PressureRef)  "<PressureRef>"
  SpeedControl1/1(ContolTorque) -> ControlTorqueLoad/1
  SpeedControllerReset/1 -> SpeedControl1/3(SpeedControllerReset)

== system windEmulatorStep4_WECSim/hptoSim/hptoModel/ControlAlgorithm/PressureBelowPmin ==
  ActualSignals : Inport
  RefValues : Inport  Port=2
  SpeedControllerReset : Inport  Port=3
  Bus Selector : BusSelector  OutputSignals=TorqueShaftInput,Pressure,wShaft
  Bus Selector1 : BusSelector  OutputSignals=TorqueInputRef,PressureRef,SheftSpeedRef
  PressureControl1 : Subsystem
  SpeedControl1 : Subsystem
  TorqueControl1 : Subsystem
  ControlSignal1 : Outport
  ControlSignal2 : Outport  Port=2
  ControlTorqueLoad : Outport  Port=3
  wires:
  ActualSignals/1 -> Bus Selector/1
  Bus Selector/1 -> TorqueControl1/1(ActualTorqueInput)  "<TorqueShaftInput>"
  TorqueControl1/1(ControlSignal1) -> ControlSignal1/1
  PressureControl1/1(ControlSignal2) -> ControlSignal2/1
  Bus Selector/2 -> TorqueControl1/3(Pressure), PressureControl1/1(ActualPressure)  "<Pressure>"
  Bus Selector/3 -> SpeedControl1/1(ShaftSpeedMotor)  "<wShaft>"
  SpeedControl1/1(ContolTorque) -> ControlTorqueLoad/1
  RefValues/1 -> Bus Selector1/1
  Bus Selector1/1 -> TorqueControl1/2(TorqueRef)  "<TorqueInputRef>"
  Bus Selector1/2 -> PressureControl1/2(PressureRef)  "<PressureRef>"
  Bus Selector1/3 -> SpeedControl1/2(ShaftSpeedRef)  "<SheftSpeedRef>"
  SpeedControllerReset/1 -> SpeedControl1/3(SpeedControllerReset)

== system windEmulatorStep4_WECSim/hptoSim/hptoModel/HPTO/ChargeCircuit ==
  note: Pressure compensated charge pump
  Check Valve1 : sh_lib/Valves/Directional Valves/Check Valve  area_max=1e-2 m^2  pres_crack=2 bar  pres_max=4 bar  C_d=0.7  A_leak=1e-12 m^2  lam_spec=1  B_lam=0.999  Re_cr=12  dynamic=0  tau=0.1 s  area_init=1e-12 m^2
      settings: InternalSimscapePortConfiguration="{\"Bottom\":[],\"Left\":[{\"id\":\"A\",\"label\":\"A\",\"type\":\"foundation.hydraulic.hydraulic\"}],\"Right\":[{\"id\":\"B\",\"label\":\"B\",\"type\":\"foundation.hydraulic.hydraulic\"}],\"Top\":[]}"
  Constant1 : Constant  Value=2000*rpm2radps
  Gas-Charged Accumulator2 : sh_lib/Accumulators/Gas-Charged Accumulator  capacity=5e-3 m^3  dead_volume=4e-5 m^3  pr_preload=100 psi  k_sh=1.4  stiff_coeff=1e10 Pa/m^3  penetr_coeff=1e10 Pa*s/m^6  flow_rate_specify=off  flow_rate_priority=None  flow_rate=5e-3 m^3/s  flow_rate_nominal_specify=off  flow_rate_nominal_value=1  flow_rate_nominal_unit=m^3/s  liquid_volume_specify=on  liquid_volume_priority=High  liquid_volume=4.9e-3 m^3  liquid_volume_nominal_specify=off  liquid_volume_nominal_value=1  liquid_volume_nominal_unit=m^3  liquid_pressure_specify=on  liquid_pressure_priority=High  liquid_pressure=400 psi  liquid_pressure_nominal_specify=off  liquid_pressure_nominal_value=1  liquid_pressure_nominal_unit=Pa
      settings: InternalSimscapePortConfiguration="{\"Bottom\":[],\"Left\":[],\"Right\":[{\"id\":\"A\",\"label\":\"A\",\"type\":\"foundation.hydraulic.hydraulic\"}],\"Top\":[]}"
  Ideal Angular Velocity Source : fl_lib/Mechanical/Mechanical Sources/Ideal Angular Velocity Source
  Mechanical Rotational Reference : fl_lib/Mechanical/Rotational Elements/Mechanical Rotational Reference
  Pressure Relief Valve2 : sh_lib/Valves/Pressure Control Valves/Pressure Relief Valve  valve_area_spec=1  p_diff_TLU=[30.15e5 : 15e3 : 31.35e5] Pa  area_TLU=[1 : 1 : 9] .* 1e-5 m^2  area_max=1e-4 m^2  pres_set=30 bar  reg_range=1 bar  C_d=0.7  A_leak=1e-12 m^2  lam_spec=1  B_lam=0.999  Re_cr=12  dynamic=0  tau=0.1 s  area_init=1e-12 m^2
      settings: InternalSimscapePortConfiguration="{\"Bottom\":[],\"Left\":[{\"id\":\"A\",\"label\":\"A\",\"type\":\"foundation.hydraulic.hydraulic\"}],\"Right\":[{\"id\":\"B\",\"label\":\"B\",\"type\":\"foundation.hydraulic.hydraulic\"}],\"Top\":[]}"
  Rate Limiter : RateLimiter  RisingSlewLimit=200  FallingSlewLimit=-200  SampleTimeMode=inherited
  Simulink-PS Converter1 : nesl_utility/Simulink-PS Converter  PhysicalDomain=network_engine_domain  SubClassName=ps_input  LeftPortType=input  RightPortType=output  PseudoPeriodic=off  Frequencies=[]  NoiseDistribution=none  NoiseParameters=[]  Unit=1  AffineConversion=off  FilteringAndDerivatives=provide  SimscapeFilterOrder=1  InputFilterTimeConstant=0.001  UdotUserProvided=0
  Variable-Displacement Pressure-Compensated Pump1 : sh_lib/Pumps and Motors/Variable-Displacement Pressure-Compensated Pump  D_max=0.2 l/rev  pr_set=20 bar  pr_reg=1 bar  efficiency_vol=0.85  efficiency_tot=0.75  pr_nominal=20 bar  w_nominal=1800 rpm  visc_nominal=18 cSt  dens_nominal=950 kg/m^3
      settings: InternalSimscapePortConfiguration="{\"Bottom\":[],\"Left\":[{\"id\":\"S\",\"label\":\"S\",\"type\":\"foundation.mechanical.rotational.rotational\"}],\"Right\":[{\"id\":\"P\",\"label\":\"P\",\"type\":\"foundation.hydraulic.hydraulic\"},{\"id\":\"T\",\"label\":\"T\",\"type\":\"foundation.hydraulic.hydraulic\"}],\"Top\":[]}"
  Conn1 : PMIOPort  Side=Left
  Conn2 : PMIOPort  Port=2  Side=Right
  wires:
  Rate Limiter/1 -> Simulink-PS Converter1/1
  Constant1/1 -> Rate Limiter/1
  connections:
  Variable-Displacement Pressure-Compensated Pump1/RConn2 -- Pressure Relief Valve2/RConn1 -- Conn2/RConn1
  Variable-Displacement Pressure-Compensated Pump1/RConn1 -- Gas-Charged Accumulator2/RConn1 -- Check Valve1/LConn1 -- Pressure Relief Valve2/LConn1
  Simulink-PS Converter1/RConn1 -- Ideal Angular Velocity Source/RConn1
  Ideal Angular Velocity Source/RConn2 -- Mechanical Rotational Reference/LConn1
  Variable-Displacement Pressure-Compensated Pump1/LConn1 -- Ideal Angular Velocity Source/LConn1
  Conn1/RConn1 -- Check Valve1/RConn1

== system windEmulatorStep4_WECSim/hptoSim/hptoModel/HPTO/FlowSensor ==
  Hydraulic Flow Rate Sensor : fl_lib/Hydraulic/Hydraulic Sensors/Hydraulic Flow Rate Sensor
  PS Terminator : fl_lib/Physical Signals/Sinks/PS Terminator
  PS-Simulink Converter : nesl_utility/PS-Simulink Converter  PhysicalDomain=network_engine_domain  SubClassName=ps_output  LeftPortType=input  RightPortType=output  PseudoPeriodic=off  Frequencies=[]  VectorFormat=1-D array  Unit=inherit  AffineConversion=off
  Scope : Scope
  m3toL : Gain  Gain=1000*60
  Qin : PMIOPort  Side=Left
  Qout : PMIOPort  Port=2  Side=Right
  FlowPump1 : Outport
  wires:
  PS-Simulink Converter/1 -> m3toL/1, Scope/1
  m3toL/1 -> FlowPump1/1  "FlowPump1"
  connections:
  PS-Simulink Converter/LConn1 -- Hydraulic Flow Rate Sensor/RConn1
  Hydraulic Flow Rate Sensor/RConn2 -- Qout/RConn1
  PS Terminator/LConn1 -- Hydraulic Flow Rate Sensor/RConn3
  Hydraulic Flow Rate Sensor/LConn1 -- Qin/RConn1

== system windEmulatorStep4_WECSim/hptoSim/hptoModel/HPTO/FlowSensor1 ==
  Gain : Gain  Gain=1000*60
  Hydraulic Flow Rate Sensor : fl_lib/Hydraulic/Hydraulic Sensors/Hydraulic Flow Rate Sensor
  PS Terminator : fl_lib/Physical Signals/Sinks/PS Terminator
  PS-Simulink Converter : nesl_utility/PS-Simulink Converter  PhysicalDomain=network_engine_domain  SubClassName=ps_output  LeftPortType=input  RightPortType=output  PseudoPeriodic=off  Frequencies=[]  VectorFormat=1-D array  Unit=inherit  AffineConversion=off
  Scope : Scope
  Qin : PMIOPort  Side=Left
  Qout : PMIOPort  Port=2  Side=Right
  wires:
  PS-Simulink Converter/1 -> Gain/1
  Gain/1 -> Scope/1  "FlowAccumulator"
  connections:
  PS-Simulink Converter/LConn1 -- Hydraulic Flow Rate Sensor/RConn1
  Hydraulic Flow Rate Sensor/RConn2 -- Qout/RConn1
  PS Terminator/LConn1 -- Hydraulic Flow Rate Sensor/RConn3
  Hydraulic Flow Rate Sensor/LConn1 -- Qin/RConn1

== system windEmulatorStep4_WECSim/hptoSim/hptoModel/HPTO/FlowSensor2 ==
  Gain : Gain  Gain=1000*60
  Hydraulic Flow Rate Sensor : fl_lib/Hydraulic/Hydraulic Sensors/Hydraulic Flow Rate Sensor
  PS Terminator : fl_lib/Physical Signals/Sinks/PS Terminator
  PS-Simulink Converter : nesl_utility/PS-Simulink Converter  PhysicalDomain=network_engine_domain  SubClassName=ps_output  LeftPortType=input  RightPortType=output  PseudoPeriodic=off  Frequencies=[]  VectorFormat=1-D array  Unit=inherit  AffineConversion=off
  Qin : PMIOPort  Side=Left
  Qout : PMIOPort  Port=2  Side=Right
  HMFlow_lpm : Outport
  wires:
  PS-Simulink Converter/1 -> Gain/1
  Gain/1 -> HMFlow_lpm/1  "FlowMotor1"
  connections:
  PS-Simulink Converter/LConn1 -- Hydraulic Flow Rate Sensor/RConn1
  Hydraulic Flow Rate Sensor/RConn2 -- Qout/RConn1
  PS Terminator/LConn1 -- Hydraulic Flow Rate Sensor/RConn3
  Hydraulic Flow Rate Sensor/LConn1 -- Qin/RConn1

== system windEmulatorStep4_WECSim/hptoSim/hptoModel/HPTO/LinearVelInput ==
  Fexc : Inport
  Ideal Force Sensor1 : fl_lib/Mechanical/Mechanical Sensors/Ideal Force Sensor
  PS-Simulink Converter : nesl_utility/PS-Simulink Converter  PhysicalDomain=network_engine_domain  SubClassName=ps_output  LeftPortType=input  RightPortType=output  PseudoPeriodic=off  Frequencies=[]  VectorFormat=1-D array  Unit=inherit  AffineConversion=off
  Subsystem : Subsystem
      settings: PortSchema="{\"entries\":[{\"content\":{\"sides\":[{\"content\":{\"connectorIds\":[\"LConn1\"]},\"type\":\"ConnectorPlacement.EquallySpacedRectSide\",\"uuid\":\"215b7bca-b171-42a0-8110-3ac7d91926b2\"},{\"content\":{\"connectorIds\":[\"RConn1\"],\"side\":\"RIGHT\"},\"type\":\"ConnectorPlacement.EquallySpacedRectSide\",\"uuid\":\"231e152d-bce3-44d9-a550-7c1231ef5d98\"},{\"content\":{\"connectorIds\":[],\"side\":\"TOP\"},\"type\":\"ConnectorPlacement.EquallySpacedRectSide\",\"uuid\":\"bc851d42-4603-42fa-9c49-ea05891b2ab9\"},{\"content\":{\"connectorIds\":[\"Out1\"],\"side\":\"BOTTOM\"},\"type\":\"ConnectorPlacement.EquallySpacedRectSide\",\"uuid\":\"67c0fa27-8a6c-4f46-81b7-2dea8cbe6936\"}]},\"type\":\"ConnectorPlacement.EquallySpacedConnector\",\"uuid\":\"7442d2b0-500a-4e34-82e4-4fa764ec5830\"}],\"packageUris\":[\"http://schema.mathworks.com/mf0/Connector/R2020b\"],\"version\":\"1.0\"}"
  WavebotModel : Subsystem
  Wheel and Axle : fl_lib/Mechanical/Mechanisms/Wheel and Axle  R=(A*2*pi/T)/targetOmega m  or=1  t_specify=off  t_priority=None  t=0 N*m  t_nominal_specify=off  t_nominal_value=1  t_nominal_unit=N*m  f_specify=off  f_priority=None  f=0 N  f_nominal_specify=off  f_nominal_value=1  f_nominal_unit=N
  Shaft : PMIOPort  Side=Left
  Output : Outport
  wires:
  Subsystem/1(LinearInput) -> Output/1
  PS-Simulink Converter/1 -> WavebotModel/1(PTOForce)
  Fexc/1 -> WavebotModel/2(Fexc)
  connections:
  PS-Simulink Converter/LConn1 -- Ideal Force Sensor1/RConn2
  WavebotModel/RConn1 -- Ideal Force Sensor1/RConn1
  Subsystem/LConn1 -- Ideal Force Sensor1/LConn1
  Wheel and Axle/RConn1 -- Subsystem/RConn1
  Wheel and Axle/LConn1 -- Shaft/RConn1

== system windEmulatorStep4_WECSim/hptoSim/hptoModel/HPTO/PressureSensor ==
  Gain : Gain  Gain=1/6894.75
  Hydraulic Pressure Sensor : fl_lib/Hydraulic/Hydraulic Sensors/Hydraulic Pressure Sensor
  Hydraulic Reference2 : fl_lib/Hydraulic/Hydraulic Elements/Hydraulic Reference
  PS-Simulink Converter : nesl_utility/PS-Simulink Converter  PhysicalDomain=network_engine_domain  SubClassName=ps_output  LeftPortType=input  RightPortType=output  PseudoPeriodic=off  Frequencies=[]  VectorFormat=1-D array  Unit=inherit  AffineConversion=off
  Scope : Scope
  P : PMIOPort  Side=Left
  Pressure : Outport
  wires:
  PS-Simulink Converter/1 -> Gain/1
  Gain/1 -> Pressure/1, Scope/1  "Pressure"
  connections:
  PS-Simulink Converter/LConn1 -- Hydraulic Pressure Sensor/RConn2
  Hydraulic Reference2/LConn1 -- Hydraulic Pressure Sensor/RConn1
  Hydraulic Pressure Sensor/LConn1 -- P/RConn1

== system windEmulatorStep4_WECSim/hptoSim/hptoModel/HPTO/Subsystem1 ==
  In1 : Inport
  Gain : Gain  Gain=0.0075
  LTI System2 : cstblocks/LTI System  sys=tf(100*2*pi,[1 200*pi])  IC=[]  PadeOrder=0
  Out1 : Outport
  wires:
  LTI System2/1 -> Gain/1
  In1/1 -> LTI System2/1
  Gain/1 -> Out1/1

== system windEmulatorStep4_WECSim/hptoSim/hptoModel/HPTO/Subsystem2 ==
  1 : Inport
  Gain : Gain  Gain=0.0075
  LTI System2 : cstblocks/LTI System  sys=tf(100*2*pi,[1 200*pi])  IC=[]  PadeOrder=0
  Out1 : Outport
  wires:
  LTI System2/1 -> Gain/1
  1/1 -> LTI System2/1
  Gain/1 -> Out1/1

== system windEmulatorStep4_WECSim/hptoSim/hptoModel/HPTO/Subsystem3 ==
  Gain : Gain  Gain=radps2rpm
  Ideal Rotational Motion Sensor : fl_lib/Mechanical/Mechanical Sensors/Ideal Rotational Motion Sensor  reference=foundation.enum.MeasurementReference.difference  acceleration_port=false  velocity_port=true  position_port=true  wrap_angle=simscape.enum.onoff.off  offset=0 rad
  Ideal Torque Sensor : fl_lib/Mechanical/Mechanical Sensors/Ideal Torque Sensor
  Mechanical Rotational Reference : fl_lib/Mechanical/Rotational Elements/Mechanical Rotational Reference
  PS Terminator : fl_lib/Physical Signals/Sinks/PS Terminator
  PS-Simulink Converter : nesl_utility/PS-Simulink Converter  PhysicalDomain=network_engine_domain  SubClassName=ps_output  LeftPortType=input  RightPortType=output  PseudoPeriodic=off  Frequencies=[]  VectorFormat=1-D array  Unit=inherit  AffineConversion=off
  PS-Simulink Converter1 : nesl_utility/PS-Simulink Converter  PhysicalDomain=network_engine_domain  SubClassName=ps_output  LeftPortType=input  RightPortType=output  PseudoPeriodic=off  Frequencies=[]  VectorFormat=1-D array  Unit=inherit  AffineConversion=off
  1 : PMIOPort  Side=Left
  2 : PMIOPort  Port=2  Side=Right
  torque_Nm : Outport
  speed_rpm : Outport  Port=2
  wires:
  PS-Simulink Converter/1 -> torque_Nm/1  "TorqueInput"
  PS-Simulink Converter1/1 -> Gain/1
  Gain/1 -> speed_rpm/1  "ShaftSpeedPump"
  connections:
  Ideal Rotational Motion Sensor/LConn1 -- Ideal Torque Sensor/LConn1 -- 1/RConn1
  Mechanical Rotational Reference/LConn1 -- Ideal Rotational Motion Sensor/RConn1
  PS Terminator/LConn1 -- Ideal Rotational Motion Sensor/RConn3
  PS-Simulink Converter1/LConn1 -- Ideal Rotational Motion Sensor/RConn2
  Ideal Torque Sensor/RConn1 -- 2/RConn1
  PS-Simulink Converter/LConn1 -- Ideal Torque Sensor/RConn2

== system windEmulatorStep4_WECSim/hptoSim/hptoModel/ControlAlgorithm/ForceToTorque/DesiredForce ==
  <LinearSpeedInput> : Inport
  <LinearPositionInput> : Inport  Port=2
  Add : Sum
  Product : Product
  Product1 : Product
  kDamping : Constant  Value=0
  kDampingNow : Gain
  kSpring : Constant  Value=0
  kSpringNow : Gain
  ForceD : Outport
  wires:
  Add/1 -> ForceD/1  "ForceD"
  kSpring/1 -> kSpringNow/1
  kDamping/1 -> kDampingNow/1
  Product1/1 -> Add/2
  Product/1 -> Add/1
  <LinearPositionInput>/1 -> Product1/1
  <LinearSpeedInput>/1 -> Product/2
  kDampingNow/1 -> Product/1
  kSpringNow/1 -> Product1/2

== system windEmulatorStep4_WECSim/hptoSim/hptoModel/ControlAlgorithm/PressureAbovePmin/PressureControl1 ==
  ActualPressure : Inport
  PressureRef : Inport  Port=2
  Add : Sum
  Discrete-Time Integrator : DiscreteIntegrator  SampleTime=-1  ICPrevOutput=DiscIntNeverNeededParam  ICPrevScaledInput=DiscIntNeverNeededParam
  Gain : Gain  Gain=PressureControl.PG
  Gain1 : Gain  Gain=PressureControl.IG
  Saturation : Saturate  UpperLimit=1  LowerLimit=-1
  Sum : Sum  Inputs=|-+
  ControlSignal2 : Outport
  wires:
  PressureRef/1 -> Sum/1
  ActualPressure/1 -> Sum/2
  Sum/1 -> Discrete-Time Integrator/1, Gain/1
  Gain/1 -> Add/1
  Discrete-Time Integrator/1 -> Gain1/1
  Gain1/1 -> Add/2
  Saturation/1 -> ControlSignal2/1
  Add/1 -> Saturation/1

== system windEmulatorStep4_WECSim/hptoSim/hptoModel/ControlAlgorithm/PressureAbovePmin/SpeedControl1 ==
  ShaftSpeedMotor : Inport
  ShaftSpeedRef : Inport  Port=2
  SpeedControllerReset : Inport  Port=3
  DeadBandController : Constant  Value=deadBandController  OutDataTypeStr=boolean
  Rate Limiter : RateLimiter  RisingSlewLimit=deadbandTorqueSlewRate  FallingSlewLimit=-deadbandTorqueSlewRate  SampleTimeMode=inherited
  Rate Limiter1 : RateLimiter  RisingSlewLimit=50  FallingSlewLimit=-50  SampleTimeMode=inherited
  Subsystem : Subsystem
  Subsystem1 : Subsystem
  Switch : Switch  Criteria=u2 > Threshold  SaturateOnIntegerOverflow=off  InputSameDT=off
  shaftSpeedRefMin : Constant  Value=0
  ContolTorque : Outport
  wires:
  ShaftSpeedRef/1 -> Subsystem/1(shaftSpeedRef), Subsystem1/2(ShaftSpeedRefMax)
  ShaftSpeedMotor/1 -> Subsystem1/1(ShaftSpeed), Subsystem/2(shaftSpeedMotor)
  SpeedControllerReset/1 -> Subsystem/3(Reset)
  shaftSpeedRefMin/1 -> Rate Limiter1/1
  Switch/1 -> ContolTorque/1
  DeadBandController/1 -> Switch/2
  Subsystem1/1(ControlTorque_Nm) -> Rate Limiter/1
  Subsystem/1(ContolTorque_Nm) -> Switch/3
  Rate Limiter/1 -> Switch/1
  Rate Limiter1/1 -> Subsystem1/3(ShaftSpeedRefMin)

== system windEmulatorStep4_WECSim/hptoSim/hptoModel/ControlAlgorithm/PressureAbovePmin/TorqueControl1 ==
  TorqueRef : Inport
  Constant : Constant  Value=-1
  Constant1 : Constant
  Switch : Switch  SaturateOnIntegerOverflow=off  InputSameDT=off
  ControlSignal1 : Outport
  wires:
  TorqueRef/1 -> Switch/2
  Constant/1 -> Switch/1
  Constant1/1 -> Switch/3
  Switch/1 -> ControlSignal1/1

== system windEmulatorStep4_WECSim/hptoSim/hptoModel/ControlAlgorithm/PressureBelowPmin/PressureControl1 ==
  ActualPressure : Inport
  PressureRef : Inport  Port=2
  Add : Sum
  Discrete-Time Integrator : DiscreteIntegrator  SampleTime=-1  ICPrevOutput=DiscIntNeverNeededParam  ICPrevScaledInput=DiscIntNeverNeededParam
  Gain : Gain  Gain=PressureControl.PG
  Gain1 : Gain  Gain=PressureControl.IG
  Saturation : Saturate  UpperLimit=1  LowerLimit=-1
  Sum : Sum  Inputs=|-+
  ControlSignal2 : Outport
  wires:
  PressureRef/1 -> Sum/1
  ActualPressure/1 -> Sum/2
  Sum/1 -> Discrete-Time Integrator/1, Gain/1
  Gain/1 -> Add/1
  Discrete-Time Integrator/1 -> Gain1/1
  Gain1/1 -> Add/2
  Saturation/1 -> ControlSignal2/1
  Add/1 -> Saturation/1
